simulink subsystem "dcm_orthonormalization"  (R2023b)
settings: Solver=VariableStepAuto  StartTime=0.0  StopTime=10.0  RelTol=1e-3
settings Model: Creator=pierb  LastModifiedBy=pierb

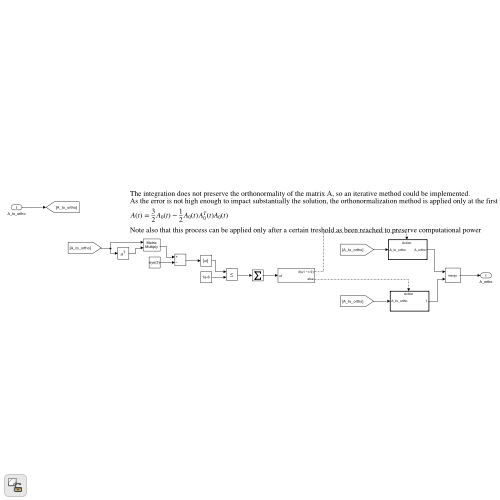
[thumbnail: Simulink's stored preview of the top-level diagram]
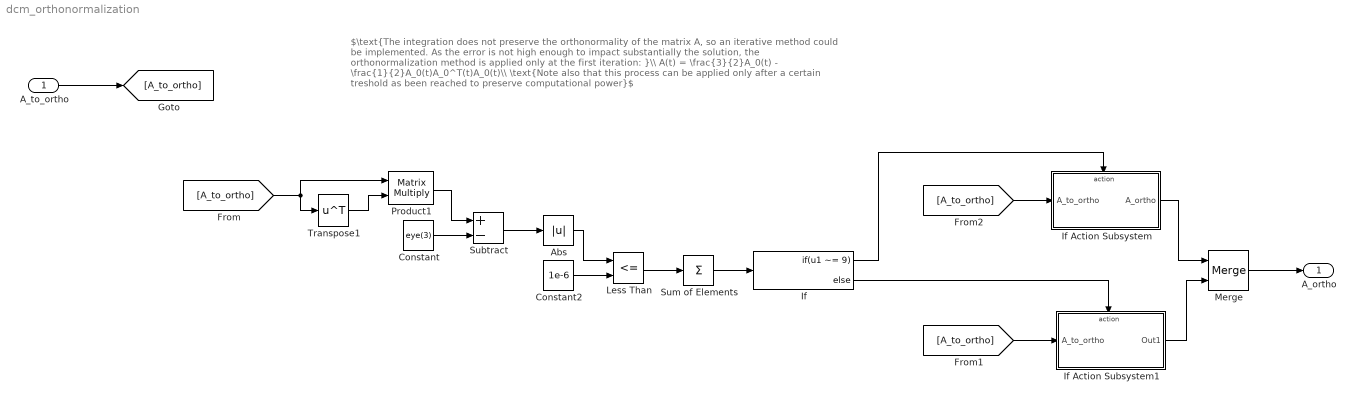
== system dcm_orthonormalization ==
  note: $\text{The integration does not preserve the orthonormality of the matrix A, so an iterative method could be implemented. As the error is not high enough to impact substantially the solution, the orthonormalization method is applied only at the first iteration: }\\ A(t) = \frac{3}{2}A_0(t) - \frac{1}{2}A_0(t)A_0^T(t)A_0(t)\\ \text{Note also that this process can be applied only after a certain treshold as been reached to preserve computational power}$
  A_to_ortho : Inport
  Abs : Abs  SaturateOnIntegerOverflow=off
  Constant : Constant  Value=eye(3)
  Constant2 : Constant  Value=1e-6
  If : If  IfExpression=u1 ~= 9
  If Action Subsystem : Subsystem  TreatAsAtomicUnit=on
  If Action Subsystem1 : Subsystem  TreatAsAtomicUnit=on
  Less Than : RelationalOperator  Operator=<=  OutDataTypeStr=boolean  RndMeth=Simplest  InputSameDT=off
  Merge : Merge
  Product1 : Product  Inputs=**  Multiplication=Matrix(*)
  Subtract : Sum  Inputs=+-
  Sum of Elements : Sum  Inputs=+
  Transpose1 : Math  Operator=transpose
  A_ortho : Outport
  wires:
  Product1/1 -> Subtract/1
  Subtract/1 -> Abs/1
  Transpose1/1 -> Product1/2
  Less Than/1 -> Sum of Elements/1
  Constant/1 -> Subtract/2
  Constant2/1 -> Less Than/2
  Abs/1 -> Less Than/1
  Sum of Elements/1 -> If/1
  If/1 -> If Action Subsystem/Action
  If/2 -> If Action Subsystem1/Action
  If Action Subsystem/1(A_ortho) -> Merge/1
  If Action Subsystem1/1(Out1) -> Merge/2
  Merge/1 -> A_ortho/1
  A_to_ortho/1 -> [A_to_ortho]
  [A_to_ortho] -> Transpose1/1, Product1/1
  [A_to_ortho] -> If Action Subsystem1/1(A_to_ortho)
  [A_to_ortho] -> If Action Subsystem/1(A_to_ortho)

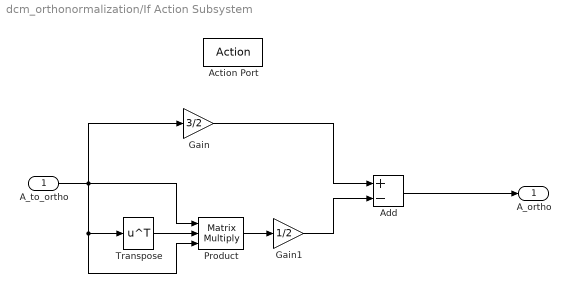
== system dcm_orthonormalization/If Action Subsystem ==
  A_to_ortho : Inport
  Action Port : ActionPort
  Add : Sum  Inputs=+-
  Gain : Gain  Gain=3/2
  Gain1 : Gain  Gain=1/2
  Product : Product  Inputs=***  Multiplication=Matrix(*)
  Transpose : Math  Operator=transpose
  A_ortho : Outport
  wires:
  Add/1 -> A_ortho/1
  Product/1 -> Gain1/1
  A_to_ortho/1 -> Gain/1, Product/1, Transpose/1, Product/3
  Transpose/1 -> Product/2
  Gain1/1 -> Add/2
  Gain/1 -> Add/1

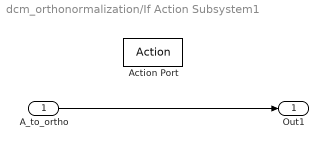
== system dcm_orthonormalization/If Action Subsystem1 ==
  A_to_ortho : Inport
  Action Port : ActionPort
  Out1 : Outport
  wires:
  A_to_ortho/1 -> Out1/1
